simulink model "lane_change_straight"  (R2018b)
settings: Solver=ode8  StartTime=0.0  StopTime=30  FixedStep=dt  RelTol=1e-3
values from neighbouring files (symbols this model uses):
  ego_dist = 0    [runsim.m]
  ego_distlat = 0    [runsim.m]
  ego_distlatc = ego_distlat + 12    (= 12)    [runsim.m]
  ego_vel = 60*mph2fps    (= 88.2)    [runsim.m]
  ego_velc = 65*mph2fps    (= 95.55)    [runsim.m]
  ego_velc2 = 60*mph2fps    (= 88.2)    [runsim.m]
  fps2mph = 1/mph2fps    (= 0.680272108844)    [requirement_lon.m]    (also in runsim.m)
  front_dist = front_safe_distance + front_dist_buffer    [runsim.m]
  front_distlat = 12    [runsim.m]
  front_distlatc = front_distlat    (= 12)    [runsim.m]
  front_safe_distance = requirement_lon(front_vel) + safe_distance_margin    [runsim.m]
  front_vel = 60*mph2fps    (= 88.2)    [runsim.m]
  rear_dist = -rear_safe_distance - rear_dist_buffer    [runsim.m]
  rear_distlat = 12    [runsim.m]
  rear_distlatc = rear_distlat    (= 12)    [runsim.m]
  rear_safe_distance = requirement_lon(rear_vel) + safe_distance_margin    [runsim.m]
  rear_vel = 65*mph2fps    (= 95.55)    [runsim.m]
  rear_vel2c = 60*mph2fps    (= 88.2)    [runsim.m]
  rear_velc = rear_vel    (= 95.55)    [runsim.m]
settings Model: Creator=suvo.ganguli  LastModifiedBy=suvo.ganguli

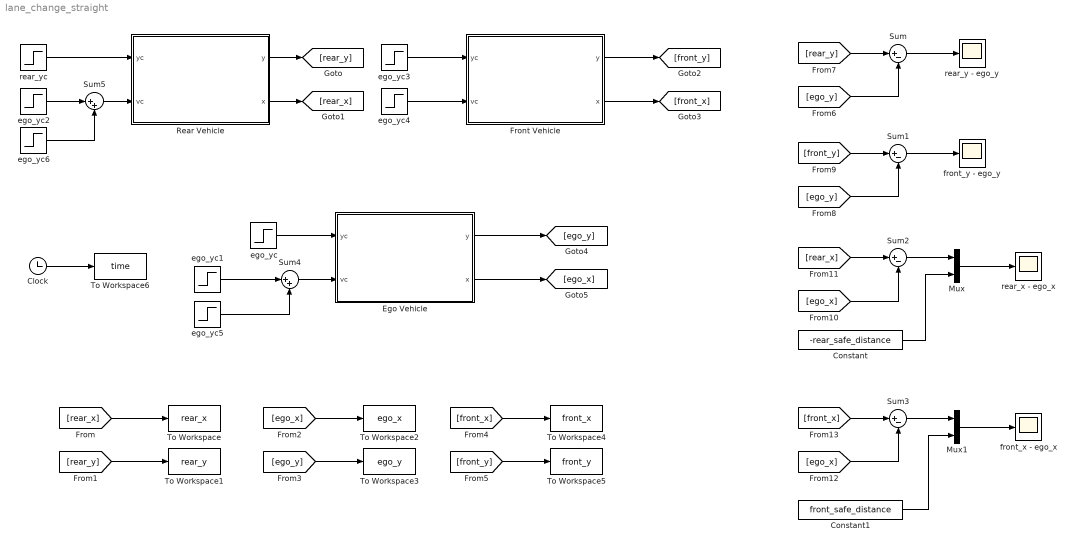
== system lane_change_straight ==
  Clock : Clock
  Constant : Constant  Value=-rear_safe_distance
  Constant1 : Constant  Value=front_safe_distance
  Ego Vehicle : Subsystem
  Front Vehicle : Subsystem
  Mux : Mux  Inputs=2
  Mux1 : Mux  Inputs=2
  Rear Vehicle : Subsystem
  Sum{,1..3} (4 alike) : Sum  Inputs=|+-
  Sum4 : Sum  Inputs=|++
  Sum5 : Sum  Inputs=|++
  To Workspace : ToWorkspace  VariableName=rear_x  SampleTime=-1
  To Workspace1 : ToWorkspace  VariableName=rear_y  SampleTime=-1
  To Workspace2 : ToWorkspace  VariableName=ego_x  SampleTime=-1
  To Workspace3 : ToWorkspace  VariableName=ego_y  SampleTime=-1
  To Workspace4 : ToWorkspace  VariableName=front_x  SampleTime=-1
  To Workspace5 : ToWorkspace  VariableName=front_y  SampleTime=-1
  To Workspace6 : ToWorkspace  VariableName=time  SampleTime=-1
  ego_yc : Step  Before=ego_dist  After=ego_distlatc  SampleTime=0
  ego_yc1 : Step  Before=ego_vel  After=ego_velc  SampleTime=0
  ego_yc2 : Step  Before=rear_vel  After=rear_velc  SampleTime=0
  ego_yc3 : Step  Before=front_distlat  After=front_distlatc  SampleTime=0
  ego_yc4 : Step  Before=front_vel  After=front_vel  SampleTime=0
  ego_yc5 : Step  Time=4  After=ego_velc2 - ego_velc  SampleTime=0
  ego_yc6 : Step  Time=4 + 2  After=rear_vel2c - rear_velc  SampleTime=0
  front_x - ego_x : Scope
  front_y - ego_y : Scope
  rear_x - ego_x : Scope
  rear_y - ego_y : Scope
  rear_yc : Step  Before=rear_distlat  After=rear_distlatc  SampleTime=0
  wires:
  rear_yc/1 -> Rear Vehicle/1(yc)
  ego_yc/1 -> Ego Vehicle/1(yc)
  ego_yc4/1 -> Front Vehicle/2(vc)
  ego_yc3/1 -> Front Vehicle/1(yc)
  Rear Vehicle/1(y) -> [rear_y]
  Rear Vehicle/2(x) -> [rear_x]
  Front Vehicle/1(y) -> [front_y]
  Front Vehicle/2(x) -> [front_x]
  Ego Vehicle/1(y) -> [ego_y]
  Ego Vehicle/2(x) -> [ego_x]
  [rear_x] -> To Workspace/1
  [rear_y] -> To Workspace1/1
  [ego_y] -> To Workspace3/1
  [ego_x] -> To Workspace2/1
  [front_x] -> To Workspace4/1
  [front_y] -> To Workspace5/1
  Sum/1 -> rear_y - ego_y/1
  [ego_y] -> Sum/2
  [rear_y] -> Sum/1
  [front_y] -> Sum1/1
  [ego_y] -> Sum1/2
  Sum1/1 -> front_y - ego_y/1
  [ego_x] -> Sum3/2
  [front_x] -> Sum3/1
  [rear_x] -> Sum2/1
  [ego_x] -> Sum2/2
  ego_yc1/1 -> Sum4/1
  ego_yc5/1 -> Sum4/2
  Sum4/1 -> Ego Vehicle/2(vc)
  Sum5/1 -> Rear Vehicle/2(vc)
  ego_yc2/1 -> Sum5/1
  ego_yc6/1 -> Sum5/2
  Sum2/1 -> Mux/1
  Mux/1 -> rear_x - ego_x/1
  Sum3/1 -> Mux1/1
  Mux1/1 -> front_x - ego_x/1
  Constant/1 -> Mux/2
  Constant1/1 -> Mux1/2
  Clock/1 -> To Workspace6/1

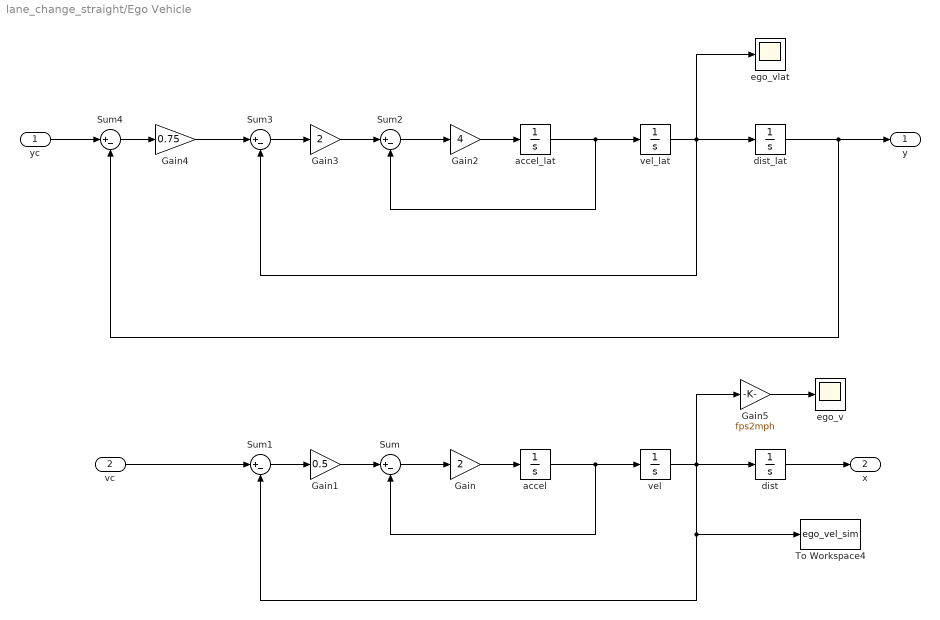
== system lane_change_straight/Ego Vehicle ==
  yc : Inport
  vc : Inport  Port=2
  Gain : Gain  Gain=2
  Gain1 : Gain  Gain=0.5
  Gain2 : Gain  Gain=4
  Gain3 : Gain  Gain=2
  Gain4 : Gain  Gain=0.75
  Gain5 : Gain  Gain=fps2mph
  Sum{,1..4} (5 alike) : Sum  Inputs=|+-
  To Workspace4 : ToWorkspace  VariableName=ego_vel_sim  SampleTime=-1
  accel : Integrator
  accel_lat : Integrator
  dist : Integrator  InitialCondition=ego_dist
  dist_lat : Integrator  InitialCondition=ego_distlat
  ego_v : Scope
  ego_vlat : Scope
  vel : Integrator  InitialCondition=ego_vel
  vel_lat : Integrator
  y : Outport
  x : Outport  Port=2
  wires:
  accel/1 -> vel/1, Sum/2
  dist/1 -> x/1
  Gain/1 -> accel/1
  Sum/1 -> Gain/1
  vel/1 -> Gain5/1, dist/1, To Workspace4/1, Sum1/2
  Gain1/1 -> Sum/1
  Sum1/1 -> Gain1/1
  vc/1 -> Sum1/1
  Gain2/1 -> accel_lat/1
  Sum2/1 -> Gain2/1
  vel_lat/1 -> ego_vlat/1, dist_lat/1, Sum3/2
  accel_lat/1 -> vel_lat/1, Sum2/2
  Sum3/1 -> Gain3/1
  Gain3/1 -> Sum2/1
  Gain4/1 -> Sum3/1
  Sum4/1 -> Gain4/1
  yc/1 -> Sum4/1
  dist_lat/1 -> Sum4/2, y/1
  Gain5/1 -> ego_v/1

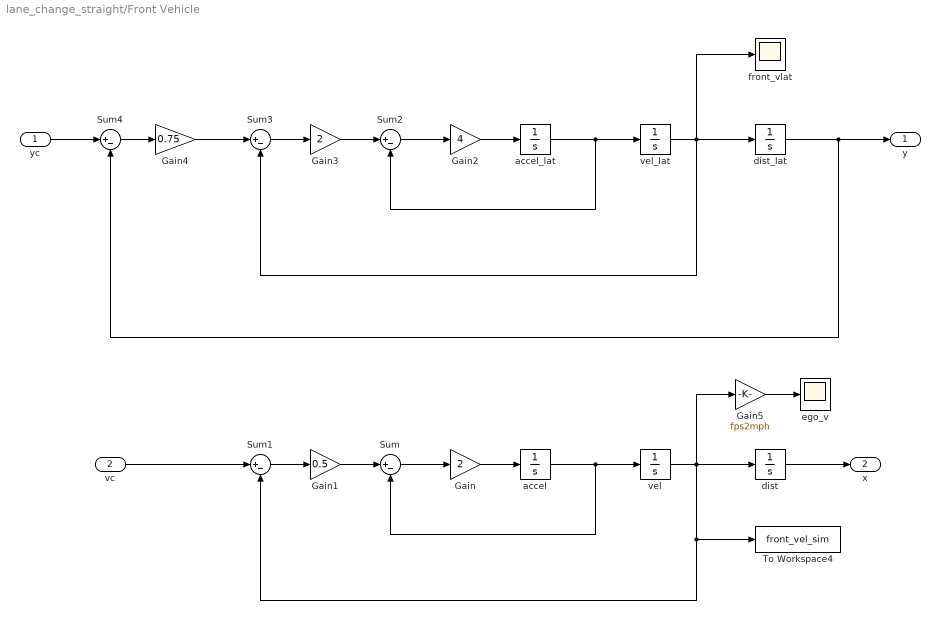
== system lane_change_straight/Front Vehicle ==
  yc : Inport
  vc : Inport  Port=2
  Gain : Gain  Gain=2
  Gain1 : Gain  Gain=0.5
  Gain2 : Gain  Gain=4
  Gain3 : Gain  Gain=2
  Gain4 : Gain  Gain=0.75
  Gain5 : Gain  Gain=fps2mph
  Sum{,1..4} (5 alike) : Sum  Inputs=|+-
  To Workspace4 : ToWorkspace  VariableName=front_vel_sim  SampleTime=-1
  accel : Integrator
  accel_lat : Integrator
  dist : Integrator  InitialCondition=front_dist
  dist_lat : Integrator  InitialCondition=front_distlat
  ego_v : Scope
  front_vlat : Scope
  vel : Integrator  InitialCondition=front_vel
  vel_lat : Integrator
  y : Outport
  x : Outport  Port=2
  wires:
  dist_lat/1 -> y/1, Sum4/2
  yc/1 -> Sum4/1
  Sum4/1 -> Gain4/1
  Gain4/1 -> Sum3/1
  Gain3/1 -> Sum2/1
  Sum3/1 -> Gain3/1
  accel_lat/1 -> Sum2/2, vel_lat/1
  vel_lat/1 -> Sum3/2, dist_lat/1, front_vlat/1
  Sum2/1 -> Gain2/1
  Gain2/1 -> accel_lat/1
  vc/1 -> Sum1/1
  Sum1/1 -> Gain1/1
  Gain1/1 -> Sum/1
  vel/1 -> To Workspace4/1, Sum1/2, dist/1, Gain5/1
  Sum/1 -> Gain/1
  Gain/1 -> accel/1
  dist/1 -> x/1
  accel/1 -> Sum/2, vel/1
  Gain5/1 -> ego_v/1

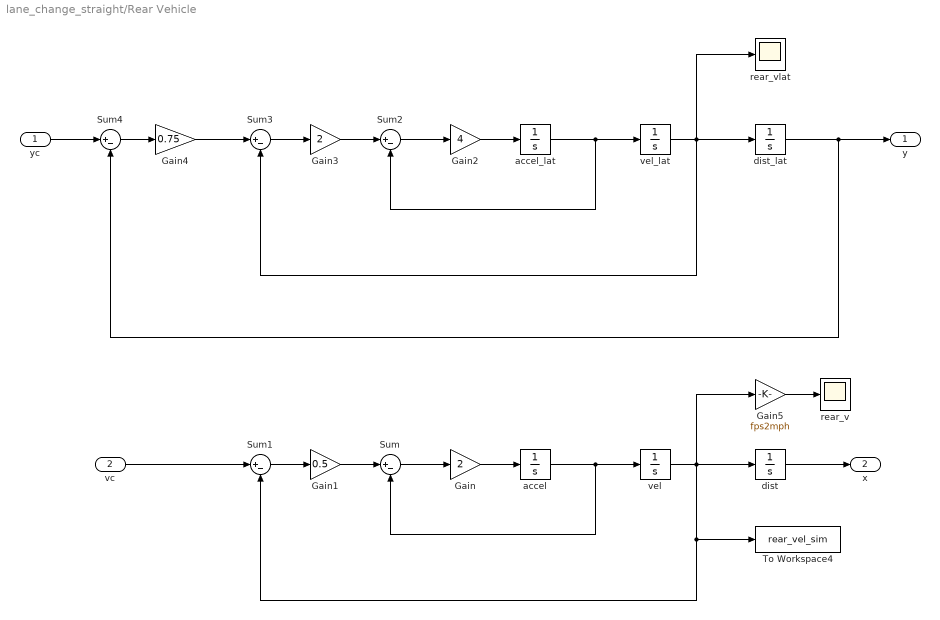
== system lane_change_straight/Rear Vehicle ==
  yc : Inport
  vc : Inport  Port=2
  Gain : Gain  Gain=2
  Gain1 : Gain  Gain=0.5
  Gain2 : Gain  Gain=4
  Gain3 : Gain  Gain=2
  Gain4 : Gain  Gain=0.75
  Gain5 : Gain  Gain=fps2mph
  Sum{,1..4} (5 alike) : Sum  Inputs=|+-
  To Workspace4 : ToWorkspace  VariableName=rear_vel_sim  SampleTime=-1
  accel : Integrator
  accel_lat : Integrator
  dist : Integrator  InitialCondition=rear_dist
  dist_lat : Integrator  InitialCondition=rear_distlat
  rear_v : Scope
  rear_vlat : Scope
  vel : Integrator  InitialCondition=rear_vel
  vel_lat : Integrator
  y : Outport
  x : Outport  Port=2
  wires:
  dist_lat/1 -> y/1, Sum4/2
  yc/1 -> Sum4/1
  Sum4/1 -> Gain4/1
  Gain4/1 -> Sum3/1
  Gain3/1 -> Sum2/1
  Sum3/1 -> Gain3/1
  accel_lat/1 -> Sum2/2, vel_lat/1
  vel_lat/1 -> Sum3/2, dist_lat/1, rear_vlat/1
  Sum2/1 -> Gain2/1
  Gain2/1 -> accel_lat/1
  vc/1 -> Sum1/1
  Sum1/1 -> Gain1/1
  Gain1/1 -> Sum/1
  vel/1 -> To Workspace4/1, Sum1/2, dist/1, Gain5/1
  Sum/1 -> Gain/1
  Gain/1 -> accel/1
  dist/1 -> x/1
  accel/1 -> Sum/2, vel/1
  Gain5/1 -> rear_v/1
